simulink model "DR18E_Testpult"  (R2017a)
settings: Solver=ode1  StartTime=0.0  StopTime=Inf  FixedStep=0.001  RelTol=1e-3
PostLoadFcn:
  | , if any(exist('dsrtsu_mdlpostloadfcn', 'file') == [2, 3, 6]), try dsrtsu_mdlpostloadfcn('Execute', bdroot); catch fprintf('Error in PostLoadFcn (dsrtsu_mdlpostloadfcn) for model "%s":\n %s\n', bdroot, lasterr); end, end,
model workspace: external: MAT-File C:\Users\DeltaRacing\Documents\dSPACE\MABX_DR18E\Model\DR18E_MABX_Parameter.mat (data not in the file)
values from neighbouring files (symbols this model uses):
  am = 1/Ts    (= 1)    [DR18E_MABX_Parameter.m]
  bm = K/Ts    (= 0.05)    [DR18E_MABX_Parameter.m]
  cf = 41350    [DR18E_MABX_Parameter.m]
  cr = 41350    [DR18E_MABX_Parameter.m]
  Derating_HV_Battery_Kapa = 1    [DR18E_MABX_Parameter.m]
  Derating_Start_km = 16    [DR18E_MABX_Parameter.m]
  Drive_Mode = 0    [DR18E_MABX_Parameter.m]
  g = 1    [DR18E_MABX_Parameter.m]
  Gas_Modus = 2    [DR18E_MABX_Parameter.m]
  HV_Power_max = 80    [DR18E_MABX_Parameter.m]
  i_Getriebe = 3.3    [DR18E_MABX_Parameter.m]
  i_Lenkgetriebe = 4.32    [DR18E_MABX_Parameter.m]
  K_SET = 1    [DR18E_MABX_Parameter.m]
  Kapazitaet_HV_Battery_kWh = 6.6    [DR18E_MABX_Parameter.m]
  KW_T_Soll = 37    [DR18E_MABX_Parameter.m]
  lf = 1.2    [DR18E_MABX_Parameter.m]
  lr = 1.15    [DR18E_MABX_Parameter.m]
  m = mdriver + mvehicle    (= 310)    [DR18E_MABX_Parameter.m]
  M_max = 150    [DR18E_MABX_Parameter.m]
  Power_Limit_onoff = 0    [DR18E_MABX_Parameter.m]
  Reifenradius = 0.2351    [DR18E_MABX_Parameter.m]
  Strecke_Endu_km = 22    [DR18E_MABX_Parameter.m]
  TC_Decr_Gas = 0.00005    (= 5e-05)    [DR18E_MABX_Parameter.m]
  TC_Derivative = 0.4    [DR18E_MABX_Parameter.m]
  TC_Incr_Gas = 0.005    [DR18E_MABX_Parameter.m]
  TC_On = 0    [DR18E_MABX_Parameter.m]
  TC_Relay_Off = 0.065    [DR18E_MABX_Parameter.m]
  TC_Relay_On = 0.07    [DR18E_MABX_Parameter.m]
  TV_Mode = 2    [DR18E_MABX_Parameter.m]
  TV_On = 0    [DR18E_MABX_Parameter.m]
  TV_Override = 1    [DR18E_MABX_Parameter.m]
  y = 0.8    [DR18E_MABX_Parameter.m]
undefined symbols (not defined in the file or in its folder): D, DiscIntNeverNeededParam, I, K_OL, P
libraries: simulink x288, rtican x100, rtiusbflightreclib x40, rti1401lib_dio_type3 x10, simulink_extras x10, rti1401lib_adc_type4 x8, rti1401lib_II_base x7
(part 27 of 27)

== system DR18E_Testpult/Eingabe Fahrzeug/BMS/Voltage Stack 1-2/Voltage Stack 2/RX Timeout Detection2/Subsystem ==
  TXStatus : Inport
  Timeout : Inport  Port=2
  Constant : Constant
  Constant1 : Constant  Value=0
  Constant2 : Constant
  Constant3 : Constant  Value=0
  Delay : Delay  DelayLength=1  InitialCondition=0
  Relational Operator : RelationalOperator  Operator=>  OutDataTypeStr=boolean  RndMeth=Nearest
  Sum : Sum  Inputs=|++
  Switch : Switch  Criteria=u2 > Threshold
  Switch1 : Switch  Criteria=u2 > Threshold
  Rampe : Outport
  RX Timeout Error : Outport  Port=2
  wires:
  TXStatus/1 -> Switch/2
  Delay/1 -> Sum/2
  Constant/1 -> Sum/1
  Sum/1 -> Switch/3
  Switch/1 -> Delay/1, Relational Operator/1, Rampe/1
  Constant1/1 -> Switch/1
  Constant2/1 -> Switch1/1
  Constant3/1 -> Switch1/3
  Switch1/1 -> RX Timeout Error/1
  Relational Operator/1 -> Switch1/2
  Timeout/1 -> Relational Operator/2

== system DR18E_Testpult/Eingabe Fahrzeug/BMS/Voltage Stack 3-4/Voltage Stack 3/RX Timeout Detection/Subsystem ==
  TXStatus : Inport
  Timeout : Inport  Port=2
  Constant : Constant
  Constant1 : Constant  Value=0
  Constant2 : Constant
  Constant3 : Constant  Value=0
  Delay : Delay  DelayLength=1  InitialCondition=0
  Relational Operator : RelationalOperator  Operator=>  OutDataTypeStr=boolean  RndMeth=Nearest
  Sum : Sum  Inputs=|++
  Switch : Switch  Criteria=u2 > Threshold
  Switch1 : Switch  Criteria=u2 > Threshold
  Rampe : Outport
  RX Timeout Error : Outport  Port=2
  wires:
  TXStatus/1 -> Switch/2
  Delay/1 -> Sum/2
  Constant/1 -> Sum/1
  Sum/1 -> Switch/3
  Switch/1 -> Delay/1, Relational Operator/1, Rampe/1
  Constant1/1 -> Switch/1
  Constant2/1 -> Switch1/1
  Constant3/1 -> Switch1/3
  Switch1/1 -> RX Timeout Error/1
  Relational Operator/1 -> Switch1/2
  Timeout/1 -> Relational Operator/2

== system DR18E_Testpult/Eingabe Fahrzeug/BMS/Voltage Stack 3-4/Voltage Stack 3/RX Timeout Detection1/Subsystem ==
  TXStatus : Inport
  Timeout : Inport  Port=2
  Constant : Constant
  Constant1 : Constant  Value=0
  Constant2 : Constant
  Constant3 : Constant  Value=0
  Delay : Delay  DelayLength=1  InitialCondition=0
  Relational Operator : RelationalOperator  Operator=>  OutDataTypeStr=boolean  RndMeth=Nearest
  Sum : Sum  Inputs=|++
  Switch : Switch  Criteria=u2 > Threshold
  Switch1 : Switch  Criteria=u2 > Threshold
  Rampe : Outport
  RX Timeout Error : Outport  Port=2
  wires:
  TXStatus/1 -> Switch/2
  Delay/1 -> Sum/2
  Constant/1 -> Sum/1
  Sum/1 -> Switch/3
  Switch/1 -> Delay/1, Relational Operator/1, Rampe/1
  Constant1/1 -> Switch/1
  Constant2/1 -> Switch1/1
  Constant3/1 -> Switch1/3
  Switch1/1 -> RX Timeout Error/1
  Relational Operator/1 -> Switch1/2
  Timeout/1 -> Relational Operator/2

== system DR18E_Testpult/Eingabe Fahrzeug/BMS/Voltage Stack 3-4/Voltage Stack 3/RX Timeout Detection2/Subsystem ==
  TXStatus : Inport
  Timeout : Inport  Port=2
  Constant : Constant
  Constant1 : Constant  Value=0
  Constant2 : Constant
  Constant3 : Constant  Value=0
  Delay : Delay  DelayLength=1  InitialCondition=0
  Relational Operator : RelationalOperator  Operator=>  OutDataTypeStr=boolean  RndMeth=Nearest
  Sum : Sum  Inputs=|++
  Switch : Switch  Criteria=u2 > Threshold
  Switch1 : Switch  Criteria=u2 > Threshold
  Rampe : Outport
  RX Timeout Error : Outport  Port=2
  wires:
  TXStatus/1 -> Switch/2
  Delay/1 -> Sum/2
  Constant/1 -> Sum/1
  Sum/1 -> Switch/3
  Switch/1 -> Delay/1, Relational Operator/1, Rampe/1
  Constant1/1 -> Switch/1
  Constant2/1 -> Switch1/1
  Constant3/1 -> Switch1/3
  Switch1/1 -> RX Timeout Error/1
  Relational Operator/1 -> Switch1/2
  Timeout/1 -> Relational Operator/2

== system DR18E_Testpult/Eingabe Fahrzeug/BMS/Voltage Stack 3-4/Voltage Stack 4/RX Timeout Detection/Subsystem ==
  TXStatus : Inport
  Timeout : Inport  Port=2
  Constant : Constant
  Constant1 : Constant  Value=0
  Constant2 : Constant
  Constant3 : Constant  Value=0
  Delay : Delay  DelayLength=1  InitialCondition=0
  Relational Operator : RelationalOperator  Operator=>  OutDataTypeStr=boolean  RndMeth=Nearest
  Sum : Sum  Inputs=|++
  Switch : Switch  Criteria=u2 > Threshold
  Switch1 : Switch  Criteria=u2 > Threshold
  Rampe : Outport
  RX Timeout Error : Outport  Port=2
  wires:
  TXStatus/1 -> Switch/2
  Delay/1 -> Sum/2
  Constant/1 -> Sum/1
  Sum/1 -> Switch/3
  Switch/1 -> Delay/1, Relational Operator/1, Rampe/1
  Constant1/1 -> Switch/1
  Constant2/1 -> Switch1/1
  Constant3/1 -> Switch1/3
  Switch1/1 -> RX Timeout Error/1
  Relational Operator/1 -> Switch1/2
  Timeout/1 -> Relational Operator/2

== system DR18E_Testpult/Eingabe Fahrzeug/BMS/Voltage Stack 3-4/Voltage Stack 4/RX Timeout Detection1/Subsystem ==
  TXStatus : Inport
  Timeout : Inport  Port=2
  Constant : Constant
  Constant1 : Constant  Value=0
  Constant2 : Constant
  Constant3 : Constant  Value=0
  Delay : Delay  DelayLength=1  InitialCondition=0
  Relational Operator : RelationalOperator  Operator=>  OutDataTypeStr=boolean  RndMeth=Nearest
  Sum : Sum  Inputs=|++
  Switch : Switch  Criteria=u2 > Threshold
  Switch1 : Switch  Criteria=u2 > Threshold
  Rampe : Outport
  RX Timeout Error : Outport  Port=2
  wires:
  TXStatus/1 -> Switch/2
  Delay/1 -> Sum/2
  Constant/1 -> Sum/1
  Sum/1 -> Switch/3
  Switch/1 -> Delay/1, Relational Operator/1, Rampe/1
  Constant1/1 -> Switch/1
  Constant2/1 -> Switch1/1
  Constant3/1 -> Switch1/3
  Switch1/1 -> RX Timeout Error/1
  Relational Operator/1 -> Switch1/2
  Timeout/1 -> Relational Operator/2

== system DR18E_Testpult/Eingabe Fahrzeug/BMS/Voltage Stack 3-4/Voltage Stack 4/RX Timeout Detection2/Subsystem ==
  TXStatus : Inport
  Timeout : Inport  Port=2
  Constant : Constant
  Constant1 : Constant  Value=0
  Constant2 : Constant
  Constant3 : Constant  Value=0
  Delay : Delay  DelayLength=1  InitialCondition=0
  Relational Operator : RelationalOperator  Operator=>  OutDataTypeStr=boolean  RndMeth=Nearest
  Sum : Sum  Inputs=|++
  Switch : Switch  Criteria=u2 > Threshold
  Switch1 : Switch  Criteria=u2 > Threshold
  Rampe : Outport
  RX Timeout Error : Outport  Port=2
  wires:
  TXStatus/1 -> Switch/2
  Delay/1 -> Sum/2
  Constant/1 -> Sum/1
  Sum/1 -> Switch/3
  Switch/1 -> Delay/1, Relational Operator/1, Rampe/1
  Constant1/1 -> Switch/1
  Constant2/1 -> Switch1/1
  Constant3/1 -> Switch1/3
  Switch1/1 -> RX Timeout Error/1
  Relational Operator/1 -> Switch1/2
  Timeout/1 -> Relational Operator/2

== system DR18E_Testpult/Eingabe Fahrzeug/BMS/Voltage Stack 5-6/Voltage Stack 5/RX Timeout Detection/Subsystem ==
  TXStatus : Inport
  Timeout : Inport  Port=2
  Constant : Constant
  Constant1 : Constant  Value=0
  Constant2 : Constant
  Constant3 : Constant  Value=0
  Delay : Delay  DelayLength=1  InitialCondition=0
  Relational Operator : RelationalOperator  Operator=>  OutDataTypeStr=boolean  RndMeth=Nearest
  Sum : Sum  Inputs=|++
  Switch : Switch  Criteria=u2 > Threshold
  Switch1 : Switch  Criteria=u2 > Threshold
  Rampe : Outport
  RX Timeout Error : Outport  Port=2
  wires:
  TXStatus/1 -> Switch/2
  Delay/1 -> Sum/2
  Constant/1 -> Sum/1
  Sum/1 -> Switch/3
  Switch/1 -> Delay/1, Relational Operator/1, Rampe/1
  Constant1/1 -> Switch/1
  Constant2/1 -> Switch1/1
  Constant3/1 -> Switch1/3
  Switch1/1 -> RX Timeout Error/1
  Relational Operator/1 -> Switch1/2
  Timeout/1 -> Relational Operator/2

== system DR18E_Testpult/Eingabe Fahrzeug/BMS/Voltage Stack 5-6/Voltage Stack 5/RX Timeout Detection1/Subsystem ==
  TXStatus : Inport
  Timeout : Inport  Port=2
  Constant : Constant
  Constant1 : Constant  Value=0
  Constant2 : Constant
  Constant3 : Constant  Value=0
  Delay : Delay  DelayLength=1  InitialCondition=0
  Relational Operator : RelationalOperator  Operator=>  OutDataTypeStr=boolean  RndMeth=Nearest
  Sum : Sum  Inputs=|++
  Switch : Switch  Criteria=u2 > Threshold
  Switch1 : Switch  Criteria=u2 > Threshold
  Rampe : Outport
  RX Timeout Error : Outport  Port=2
  wires:
  TXStatus/1 -> Switch/2
  Delay/1 -> Sum/2
  Constant/1 -> Sum/1
  Sum/1 -> Switch/3
  Switch/1 -> Delay/1, Relational Operator/1, Rampe/1
  Constant1/1 -> Switch/1
  Constant2/1 -> Switch1/1
  Constant3/1 -> Switch1/3
  Switch1/1 -> RX Timeout Error/1
  Relational Operator/1 -> Switch1/2
  Timeout/1 -> Relational Operator/2

== system DR18E_Testpult/Eingabe Fahrzeug/BMS/Voltage Stack 5-6/Voltage Stack 5/RX Timeout Detection2/Subsystem ==
  TXStatus : Inport
  Timeout : Inport  Port=2
  Constant : Constant
  Constant1 : Constant  Value=0
  Constant2 : Constant
  Constant3 : Constant  Value=0
  Delay : Delay  DelayLength=1  InitialCondition=0
  Relational Operator : RelationalOperator  Operator=>  OutDataTypeStr=boolean  RndMeth=Nearest
  Sum : Sum  Inputs=|++
  Switch : Switch  Criteria=u2 > Threshold
  Switch1 : Switch  Criteria=u2 > Threshold
  Rampe : Outport
  RX Timeout Error : Outport  Port=2
  wires:
  TXStatus/1 -> Switch/2
  Delay/1 -> Sum/2
  Constant/1 -> Sum/1
  Sum/1 -> Switch/3
  Switch/1 -> Delay/1, Relational Operator/1, Rampe/1
  Constant1/1 -> Switch/1
  Constant2/1 -> Switch1/1
  Constant3/1 -> Switch1/3
  Switch1/1 -> RX Timeout Error/1
  Relational Operator/1 -> Switch1/2
  Timeout/1 -> Relational Operator/2

== system DR18E_Testpult/Eingabe Fahrzeug/BMS/Voltage Stack 5-6/Voltage Stack 6/RX Timeout Detection/Subsystem ==
  TXStatus : Inport
  Timeout : Inport  Port=2
  Constant : Constant
  Constant1 : Constant  Value=0
  Constant2 : Constant
  Constant3 : Constant  Value=0
  Delay : Delay  DelayLength=1  InitialCondition=0
  Relational Operator : RelationalOperator  Operator=>  OutDataTypeStr=boolean  RndMeth=Nearest
  Sum : Sum  Inputs=|++
  Switch : Switch  Criteria=u2 > Threshold
  Switch1 : Switch  Criteria=u2 > Threshold
  Rampe : Outport
  RX Timeout Error : Outport  Port=2
  wires:
  TXStatus/1 -> Switch/2
  Delay/1 -> Sum/2
  Constant/1 -> Sum/1
  Sum/1 -> Switch/3
  Switch/1 -> Delay/1, Relational Operator/1, Rampe/1
  Constant1/1 -> Switch/1
  Constant2/1 -> Switch1/1
  Constant3/1 -> Switch1/3
  Switch1/1 -> RX Timeout Error/1
  Relational Operator/1 -> Switch1/2
  Timeout/1 -> Relational Operator/2

== system DR18E_Testpult/Eingabe Fahrzeug/BMS/Voltage Stack 5-6/Voltage Stack 6/RX Timeout Detection1/Subsystem ==
  TXStatus : Inport
  Timeout : Inport  Port=2
  Constant : Constant
  Constant1 : Constant  Value=0
  Constant2 : Constant
  Constant3 : Constant  Value=0
  Delay : Delay  DelayLength=1  InitialCondition=0
  Relational Operator : RelationalOperator  Operator=>  OutDataTypeStr=boolean  RndMeth=Nearest
  Sum : Sum  Inputs=|++
  Switch : Switch  Criteria=u2 > Threshold
  Switch1 : Switch  Criteria=u2 > Threshold
  Rampe : Outport
  RX Timeout Error : Outport  Port=2
  wires:
  TXStatus/1 -> Switch/2
  Delay/1 -> Sum/2
  Constant/1 -> Sum/1
  Sum/1 -> Switch/3
  Switch/1 -> Delay/1, Relational Operator/1, Rampe/1
  Constant1/1 -> Switch/1
  Constant2/1 -> Switch1/1
  Constant3/1 -> Switch1/3
  Switch1/1 -> RX Timeout Error/1
  Relational Operator/1 -> Switch1/2
  Timeout/1 -> Relational Operator/2

== system DR18E_Testpult/Eingabe Fahrzeug/BMS/Voltage Stack 5-6/Voltage Stack 6/RX Timeout Detection2/Subsystem ==
  TXStatus : Inport
  Timeout : Inport  Port=2
  Constant : Constant
  Constant1 : Constant  Value=0
  Constant2 : Constant
  Constant3 : Constant  Value=0
  Delay : Delay  DelayLength=1  InitialCondition=0
  Relational Operator : RelationalOperator  Operator=>  OutDataTypeStr=boolean  RndMeth=Nearest
  Sum : Sum  Inputs=|++
  Switch : Switch  Criteria=u2 > Threshold
  Switch1 : Switch  Criteria=u2 > Threshold
  Rampe : Outport
  RX Timeout Error : Outport  Port=2
  wires:
  TXStatus/1 -> Switch/2
  Delay/1 -> Sum/2
  Constant/1 -> Sum/1
  Sum/1 -> Switch/3
  Switch/1 -> Delay/1, Relational Operator/1, Rampe/1
  Constant1/1 -> Switch/1
  Constant2/1 -> Switch1/1
  Constant3/1 -> Switch1/3
  Switch1/1 -> RX Timeout Error/1
  Relational Operator/1 -> Switch1/2
  Timeout/1 -> Relational Operator/2

== system DR18E_Testpult/Eingabe Fahrzeug/BMS/Voltage Stack 7-8/Voltage Stack 7/RX Timeout Detection/Subsystem ==
  TXStatus : Inport
  Timeout : Inport  Port=2
  Constant : Constant
  Constant1 : Constant  Value=0
  Constant2 : Constant
  Constant3 : Constant  Value=0
  Delay : Delay  DelayLength=1  InitialCondition=0
  Relational Operator : RelationalOperator  Operator=>  OutDataTypeStr=boolean  RndMeth=Nearest
  Sum : Sum  Inputs=|++
  Switch : Switch  Criteria=u2 > Threshold
  Switch1 : Switch  Criteria=u2 > Threshold
  Rampe : Outport
  RX Timeout Error : Outport  Port=2
  wires:
  TXStatus/1 -> Switch/2
  Delay/1 -> Sum/2
  Constant/1 -> Sum/1
  Sum/1 -> Switch/3
  Switch/1 -> Delay/1, Relational Operator/1, Rampe/1
  Constant1/1 -> Switch/1
  Constant2/1 -> Switch1/1
  Constant3/1 -> Switch1/3
  Switch1/1 -> RX Timeout Error/1
  Relational Operator/1 -> Switch1/2
  Timeout/1 -> Relational Operator/2

== system DR18E_Testpult/Eingabe Fahrzeug/BMS/Voltage Stack 7-8/Voltage Stack 7/RX Timeout Detection1/Subsystem ==
  TXStatus : Inport
  Timeout : Inport  Port=2
  Constant : Constant
  Constant1 : Constant  Value=0
  Constant2 : Constant
  Constant3 : Constant  Value=0
  Delay : Delay  DelayLength=1  InitialCondition=0
  Relational Operator : RelationalOperator  Operator=>  OutDataTypeStr=boolean  RndMeth=Nearest
  Sum : Sum  Inputs=|++
  Switch : Switch  Criteria=u2 > Threshold
  Switch1 : Switch  Criteria=u2 > Threshold
  Rampe : Outport
  RX Timeout Error : Outport  Port=2
  wires:
  TXStatus/1 -> Switch/2
  Delay/1 -> Sum/2
  Constant/1 -> Sum/1
  Sum/1 -> Switch/3
  Switch/1 -> Delay/1, Relational Operator/1, Rampe/1
  Constant1/1 -> Switch/1
  Constant2/1 -> Switch1/1
  Constant3/1 -> Switch1/3
  Switch1/1 -> RX Timeout Error/1
  Relational Operator/1 -> Switch1/2
  Timeout/1 -> Relational Operator/2

== system DR18E_Testpult/Eingabe Fahrzeug/BMS/Voltage Stack 7-8/Voltage Stack 7/RX Timeout Detection2/Subsystem ==
  TXStatus : Inport
  Timeout : Inport  Port=2
  Constant : Constant
  Constant1 : Constant  Value=0
  Constant2 : Constant
  Constant3 : Constant  Value=0
  Delay : Delay  DelayLength=1  InitialCondition=0
  Relational Operator : RelationalOperator  Operator=>  OutDataTypeStr=boolean  RndMeth=Nearest
  Sum : Sum  Inputs=|++
  Switch : Switch  Criteria=u2 > Threshold
  Switch1 : Switch  Criteria=u2 > Threshold
  Rampe : Outport
  RX Timeout Error : Outport  Port=2
  wires:
  TXStatus/1 -> Switch/2
  Delay/1 -> Sum/2
  Constant/1 -> Sum/1
  Sum/1 -> Switch/3
  Switch/1 -> Delay/1, Relational Operator/1, Rampe/1
  Constant1/1 -> Switch/1
  Constant2/1 -> Switch1/1
  Constant3/1 -> Switch1/3
  Switch1/1 -> RX Timeout Error/1
  Relational Operator/1 -> Switch1/2
  Timeout/1 -> Relational Operator/2

== system DR18E_Testpult/Eingabe Fahrzeug/BMS/Voltage Stack 7-8/Voltage Stack 8/RX Timeout Detection/Subsystem ==
  TXStatus : Inport
  Timeout : Inport  Port=2
  Constant : Constant
  Constant1 : Constant  Value=0
  Constant2 : Constant
  Constant3 : Constant  Value=0
  Delay : Delay  DelayLength=1  InitialCondition=0
  Relational Operator : RelationalOperator  Operator=>  OutDataTypeStr=boolean  RndMeth=Nearest
  Sum : Sum  Inputs=|++
  Switch : Switch  Criteria=u2 > Threshold
  Switch1 : Switch  Criteria=u2 > Threshold
  Rampe : Outport
  RX Timeout Error : Outport  Port=2
  wires:
  TXStatus/1 -> Switch/2
  Delay/1 -> Sum/2
  Constant/1 -> Sum/1
  Sum/1 -> Switch/3
  Switch/1 -> Delay/1, Relational Operator/1, Rampe/1
  Constant1/1 -> Switch/1
  Constant2/1 -> Switch1/1
  Constant3/1 -> Switch1/3
  Switch1/1 -> RX Timeout Error/1
  Relational Operator/1 -> Switch1/2
  Timeout/1 -> Relational Operator/2

== system DR18E_Testpult/Eingabe Fahrzeug/BMS/Voltage Stack 7-8/Voltage Stack 8/RX Timeout Detection1/Subsystem ==
  TXStatus : Inport
  Timeout : Inport  Port=2
  Constant : Constant
  Constant1 : Constant  Value=0
  Constant2 : Constant
  Constant3 : Constant  Value=0
  Delay : Delay  DelayLength=1  InitialCondition=0
  Relational Operator : RelationalOperator  Operator=>  OutDataTypeStr=boolean  RndMeth=Nearest
  Sum : Sum  Inputs=|++
  Switch : Switch  Criteria=u2 > Threshold
  Switch1 : Switch  Criteria=u2 > Threshold
  Rampe : Outport
  RX Timeout Error : Outport  Port=2
  wires:
  TXStatus/1 -> Switch/2
  Delay/1 -> Sum/2
  Constant/1 -> Sum/1
  Sum/1 -> Switch/3
  Switch/1 -> Delay/1, Relational Operator/1, Rampe/1
  Constant1/1 -> Switch/1
  Constant2/1 -> Switch1/1
  Constant3/1 -> Switch1/3
  Switch1/1 -> RX Timeout Error/1
  Relational Operator/1 -> Switch1/2
  Timeout/1 -> Relational Operator/2

== system DR18E_Testpult/Eingabe Fahrzeug/BMS/Voltage Stack 7-8/Voltage Stack 8/RX Timeout Detection2/Subsystem ==
  TXStatus : Inport
  Timeout : Inport  Port=2
  Constant : Constant
  Constant1 : Constant  Value=0
  Constant2 : Constant
  Constant3 : Constant  Value=0
  Delay : Delay  DelayLength=1  InitialCondition=0
  Relational Operator : RelationalOperator  Operator=>  OutDataTypeStr=boolean  RndMeth=Nearest
  Sum : Sum  Inputs=|++
  Switch : Switch  Criteria=u2 > Threshold
  Switch1 : Switch  Criteria=u2 > Threshold
  Rampe : Outport
  RX Timeout Error : Outport  Port=2
  wires:
  TXStatus/1 -> Switch/2
  Delay/1 -> Sum/2
  Constant/1 -> Sum/1
  Sum/1 -> Switch/3
  Switch/1 -> Delay/1, Relational Operator/1, Rampe/1
  Constant1/1 -> Switch/1
  Constant2/1 -> Switch1/1
  Constant3/1 -> Switch1/3
  Switch1/1 -> RX Timeout Error/1
  Relational Operator/1 -> Switch1/2
  Timeout/1 -> Relational Operator/2

== system DR18E_Testpult/Eingabe Fahrzeug/Inverter Feedback Messages/Istwerte Umrichter 1 empfangen /Drehzahl/PT1 Discrete2/Subsystem ==
  T : Inport
  Constant : Constant
  Constant2 : Constant
  Divide : Product  Inputs=*/
  Divide1 : Product  Inputs=*/
  Sum : Sum  Inputs=|++
  Weighted Sample Time : SampleTimeMath  TsampMathOp=Ts Only
  T* : Outport
  wires:
  Divide1/1 -> Sum/1
  Constant2/1 -> Sum/2
  T/1 -> Divide1/1
  Sum/1 -> Divide/2
  Constant/1 -> Divide/1
  Weighted Sample Time/1 -> Divide1/2
  Divide/1 -> T*/1

== system DR18E_Testpult/Eingabe Fahrzeug/Inverter Feedback Messages/Istwerte Umrichter 2 empfangen/Drehzahl/PT1 Discrete2/Subsystem ==
  T : Inport
  Constant : Constant
  Constant2 : Constant
  Divide : Product  Inputs=*/
  Divide1 : Product  Inputs=*/
  Sum : Sum  Inputs=|++
  Weighted Sample Time : SampleTimeMath  TsampMathOp=Ts Only
  T* : Outport
  wires:
  Divide1/1 -> Sum/1
  Constant2/1 -> Sum/2
  T/1 -> Divide1/1
  Sum/1 -> Divide/2
  Constant/1 -> Divide/1
  Weighted Sample Time/1 -> Divide1/2
  Divide/1 -> T*/1

== system DR18E_Testpult/Eingabe Fahrzeug/MicroAutoBox/AI/Umrechnung Widerstand - Temperatur NTC/PT1 Discrete1/Subsystem ==
  T : Inport
  Constant : Constant
  Constant2 : Constant
  Divide : Product  Inputs=*/
  Divide1 : Product  Inputs=*/
  Sum : Sum  Inputs=|++
  Weighted Sample Time : SampleTimeMath  TsampMathOp=Ts Only
  T* : Outport
  wires:
  Divide1/1 -> Sum/1
  Constant2/1 -> Sum/2
  T/1 -> Divide1/1
  Sum/1 -> Divide/2
  Constant/1 -> Divide/1
  Weighted Sample Time/1 -> Divide1/2
  Divide/1 -> T*/1

== system DR18E_Testpult/Eingabe Fahrzeug/MicroAutoBox/AI/Umrechnung Widerstand - Temperatur NTC1/PT1 Discrete1/Subsystem ==
  T : Inport
  Constant : Constant
  Constant2 : Constant
  Divide : Product  Inputs=*/
  Divide1 : Product  Inputs=*/
  Sum : Sum  Inputs=|++
  Weighted Sample Time : SampleTimeMath  TsampMathOp=Ts Only
  T* : Outport
  wires:
  Divide1/1 -> Sum/1
  Constant2/1 -> Sum/2
  T/1 -> Divide1/1
  Sum/1 -> Divide/2
  Constant/1 -> Divide/1
  Weighted Sample Time/1 -> Divide1/2
  Divide/1 -> T*/1

== stateflow chart DR18E_Testpult/Verarbeitung/Vehicle State Machine/Fahrzeugsteuerung ==
  settings: updateMethod=DISCRETE  sampleTime=1e-3
  state Init
    en: O_Sicherheitskreis_Enable = 0;
    settings: description=|
        | Umrichter Initialisierung
        | 
        | Parametrierung der beiden Umrichter, damit Ist-Werte zyklisch gesendet werden.
    state UmrichterInit
      en: O_Inverter_TX_Mode = 1; //TX Modus: Initialisierung
      state initEntry
        en: O_State = 10;
      state U_init
        en: O_State = 11;
        en: O_U1Init_Reg = I_vecU1config_TXRegister[i];
        en: O_U1Init_Zeit = I_vecU1config_TXZeiten[i];
        en: O_U2Init_Reg = I_vecU2config_TXRegister[i];
        en: O_U2Init_Zeit = I_vecU2config_TXZeiten[i] ;
      note: For-Schleife
          | über alle
          | 8 Configs
      state wait
        en: O_State = 12;
      state CANTimeoutInit
        /*en: O_U1_RegID = 208; //0xD0
        en: O_U2_RegID = 208; //0xD0
        en: O_U1_Value32 = 1000; //Timeout in ms
        en: O_U2_Value32 = 1000; //Timeout in ms*/
        en: O_Inverter_TX_Mode = 2;
        //Universal TX Mode
        ex: O_U1_RegID = 0;
        ex: O_U1_RegID = 0;
      (default) -> initEntry
      initEntry -> (junction 759) : after(5,sec)
      (junction 759) -> (junction 211) : {i = 0;}
      (junction 211) -> U_init [order 1] : [i < 8]
      (junction 222) -> (junction 211) : {i++;}
      (junction 211) -> CANTimeoutInit [order 2]
      U_init -> wait : after(0.01,sec)
      wait -> (junction 222) : after(0.1,sec)
    state Boards_Init
      en: en: O_Inverter_TX_Mode = 2;
      //Universal TX Mode
      en: Board_Init_ok = 1;
      en: O_InvertersTXActive = 1;
      en: O_State = 16;
      en: O_coolingEnable = 0;
    state Check_Safety
      state Error_In_Flash
        en: O_AMSIMDFlash = 1;
        en: en: O_State = 18.1;
      state Safety_Error2
        en: O_ErrorNr = 6;
        en: O_State = 17.7;
        exit: e_Error;
      state Error_In_Flash_Reset
        en: O_AMSIMDFlash = 0;
        en: O_State = 18.2;
      state Safety_Error3
        en: O_ErrorNr = 7;
        en: O_State = 17.8;
        exit: e_Error;
      note: ERROR
      state Safety_Error
        en: O_ErrorNr = 2;
        en: O_State = 17.1;
        exit: e_Error;
      state Safety_Error1
        en: O_ErrorNr = 1;
        en: O_State = 17.2;
        exit: e_Error;
      state Safety_Error4
        en: O_ErrorNr = 3;
        en: O_State = 17.3;
        exit: e_Error;
      state Safety_Error5
        en: O_ErrorNr = 4;
        en: O_State = 17.4;
        exit: e_Error;
      state Safety_Error6
        en: O_ErrorNr = 5;
        en: O_State = 17.5;
        exit: e_Error;
      state Safety_Error7
        en: O_ErrorNr = 8;
        en: O_State = 17.6;
        exit: e_Error;
      state Safety_Error_Reset
        en: O_ErrorNr = 0;
        en: O_AMSIMDFlash = 0;
        en: O_State = 19;
        exit: e_Error;
      (junction 673) -> (junction 671) : after(0.2,sec)
      (default) -> (junction 671)
      Init.Check_Safety.Safety_Error2 -> Init.Check_Safety.Error_In_Flash
      (junction 671) -> Init.Check_Safety.Safety_Error2 [order 2] : [A_AMS]
      (junction 671) -> (junction 672) [order 1] : [!A_AMS]
      (junction 672) -> Init.Check_Safety.Safety_Error3 [order 1] : [A_IMD]
      Init.Check_Safety.Safety_Error3 -> Init.Check_Safety.Error_In_Flash
      (junction 672) -> (junction 674) [order 2] : [!A_IMD]
      Init.Check_Safety.Error_In_Flash_Reset -> (junction 673)
      Init.Check_Safety.Safety_Error -> (junction 673)
      Init.Check_Safety.Safety_Error4 -> (junction 673)
      Init.Check_Safety.Safety_Error7 -> (junction 673)
      Init.Check_Safety.Safety_Error6 -> (junction 673)
      Init.Check_Safety.Safety_Error5 -> (junction 673)
      Init.Check_Safety.Safety_Error1 -> (junction 673)
      Init.Check_Safety.Error_In_Flash -> Init.Check_Safety.Error_In_Flash_Reset : [I_AMS_IMD_Reset]
      (junction 674) -> Init.Check_Safety.Safety_Error [order 2] : [A_BRAKE_OVERTRAVEL]
      (junction 674) -> (junction 675) [order 1] : [!A_BRAKE_OVERTRAVEL]
      (junction 675) -> Init.Check_Safety.Safety_Error1 [order 1] : [A_BPD]
      (junction 675) -> (junction 676) [order 2] : [!A_BPD]
      (junction 676) -> Init.Check_Safety.Safety_Error4 [order 1] : [A_NOT_COCKPIT]
      (junction 676) -> (junction 677) [order 2] : [!A_NOT_COCKPIT]
      (junction 677) -> Init.Check_Safety.Safety_Error5 [order 1] : [A_NOT_LINKS]
      (junction 677) -> (junction 678) [order 2] : [!A_NOT_LINKS]
      (junction 678) -> Init.Check_Safety.Safety_Error6 [order 1] : [A_NOT_RECHTS]
      (junction 678) -> (junction 679) [order 2] : [!A_NOT_RECHTS]
      (junction 679) -> Init.Check_Safety.Safety_Error7 [order 1] : [A_HVD]
      (junction 679) -> Init.Check_Safety.Safety_Error_Reset [order 2] : [!A_HVD]
    state Blink_Start_Button
      en: O_State = 20;
      en: Init_complete = 1;
    CANTimeoutInit -> Boards_Init : after(0.1,sec)
        | /*Umrichter Init Complete*/
    (default) -> UmrichterInit
    Boards_Init -> Check_Safety
    Init.Check_Safety.Safety_Error_Reset -> Blink_Start_Button
  note: Systeminitialisierung
  state Idle
    en: O_Sicherheitskreis_Enable = 0;
    en: O_State = 21;
    en: O_fBlink_Start = 2;
    settings: description=|
        | Idle-Modus
        | 
        | GLVS ist aktiv
        | TS ist inaktiv
        | 
        | Grundzustand der Fahrzeugsteuerung. Alle Antriebssysteme sind dekativiert, AIRs sind geöffnet.
        | Verlassen des Zustands durch Drücken der Start-Taste bei gleichzeitigem Betätigen des Bremspedals.
        | 
        | In diesen Zustand wird aus allen Zuständen zurückgekehrt, sobald der Sicherheitskreis anspricht.
  state TS_init
    settings: description=|
        | TS-Init Modus
        | 
        | Initialisierung des Tractive Systems.
        | Das heißt:
        | -Precharge
        | -Prüfen ob AIRs geschlossen sind und Ziel-Ladespannung des Zwischenkreises erreicht ist
        | 
        | Zustand wird verlassen, wenn Precharge abgeschlossen, AIRs geschlossen und Ziel-Spannung erreicht ist
    note: Sicherheitskreis geschlossen
        | und Entladerelais geöffnet
    state Precharge
      du: O_fBlink_Start = 0;
      state Precharge_Prepare
        en: O_Precharge_Enable = 1;
        en: O_State = 22;
      state Precharge_Start
        en: O_Sicherheitskreis_Enable = 1;
        en: O_State = 23;
        //du: e_clearPowervoltage;
      note: Precharge startet!
      state AIR_Error4
        en: O_ErrorNr = 36;
        en: O_State = 24.1;
        exit: e_Error;
      state AIR_Error
        en: O_ErrorNr = 31;
        en: O_State = 24.2;
        exit: e_Error;
      state AIR_Error1
        en: O_ErrorNr = 32;
        en: O_State = 24.3;
        exit: e_Error;
      state Precharge_TimeError
        en: O_ErrorNr = 33;
        en: O_State = 25;
        exit: e_Error;
      state Precharge_Done
        en: O_Precharge_Enable = 0;
        en: O_ErrorNr = 0;
        en: O_State = 26;
        exit: e_Error;
      state AIR_Disable
        en: O_Sicherheitskreis_Enable = 0;
        en: O_Precharge_Enable = 0;
        en: O_State = 24.4;
      state AIR_Error2
        en: O_ErrorNr = 34;
        en: O_State = 27.1;
        exit: e_Error;
      state AIR_Error3
        en: O_ErrorNr = 35;
        en: O_State = 27.2;
        exit: e_Error;
      state AIR_Error5
        en: O_ErrorNr = 37;
        en: O_State = 27.3;
        exit: e_Error;
      note: Precharge erledigt, nun
          | Prechargerelais öffnen.
          | Pluspol  AIRs schließen
          | automatisch durch Verriegelung
          | gegen Precharge Relais
      (default) -> Precharge_Prepare
      Precharge_Prepare -> Precharge_Start : after(0.1,sec)
      Precharge_Start -> (junction 291) [order 2] : [false]
          | //after(0.5,sec)
      Precharge_Start -> (junction 290) [order 1] : //[AIR_L & AIR_Rminus]
      (junction 291) -> AIR_Error4 [order 3] : //beide Relais schalten nicht
          | [!AIR_L]
      (junction 291) -> AIR_Error [order 1] : [!AIR_L]
      (junction 291) -> AIR_Error1 [order 2] : [AIR_L]
      (junction 290) -> Precharge_Done [order 2] : //EV4.12.1
          | [I_U_Zwischenkreis >= (0.90*I_U_Batt)]
      (junction 290) -> Precharge_TimeError [order 1] : //Zu lange PrechargeZeit
          | after(15,sec)
      AIR_Error1 -> (junction 299)
      AIR_Error4 -> (junction 299)
      AIR_Error -> (junction 299)
      Precharge_TimeError -> (junction 299)
      Precharge_Done -> (junction 386) [order 1] : [false]
          | //after(0.5,sec)
      (junction 299) -> AIR_Disable
      AIR_Error5 -> (junction 299)
      AIR_Error3 -> (junction 299)
      AIR_Error2 -> (junction 299)
      (junction 386) -> AIR_Error2 [order 1] : [AIR_R]
      (junction 386) -> AIR_Error5 [order 3] : //beide AIRs schließen nicht
          | [!AIR_R]
      (junction 386) -> AIR_Error3 [order 2] : [!AIR_R]
    note: TODO:
        | Error Handling
    state ClearPowervoltageError
      /*en: O_U1_RegID = 143; //0x8F
      en: O_U2_RegID = 143; //0x8F
      en: O_U1_Value32 = 0;
      en: O_U2_Value32 = 0;
      en: O_Inverter_TX_Mode = 2; //Universal TX Mode
      ex: O_U1_RegID = 0;
      ex: O_U1_RegID = 0;*/
    (default) -> Precharge
    Precharge_Done -> ClearPowervoltageError [order 2] : //Precharge OK
        | [AIR_R]
  state Check_Safety1
    en: O_Sicherheitskreis_Enable = 0;
    en: O_Precharge_Enable = 0
    en: O_fBlink_Start = 0;
    state Error_In_Flash
      en: O_AMSIMDFlash = 1;
      en: en: O_State = 48.1;
    state Safety_Error2
      en: O_ErrorNr = 6;
      en: O_State = 47.7;
      exit: e_Error;
    state Error_In_Flash_Reset
      en: O_AMSIMDFlash = 0;
      en: O_State = 48.2;
    state Safety_Error3
      en: O_ErrorNr = 7;
      en: O_State = 47.8;
      exit: e_Error;
    state Safety_Error
      en: O_ErrorNr = 2;
      en: O_State = 47.1;
      exit: e_Error;
    state Safety_Error1
      en: O_ErrorNr = 1;
      en: O_State = 47.2;
      exit: e_Error;
    state Safety_Error4
      en: O_ErrorNr = 3;
      en: O_State = 47.3;
      exit: e_Error;
    state Safety_Error5
      en: O_ErrorNr = 4;
      en: O_State = 47.4;
      exit: e_Error;
    state Safety_Error6
      en: O_ErrorNr = 5;
      en: O_State = 47.5;
      exit: e_Error;
    state Safety_Error7
      en: O_ErrorNr = 8;
      en: O_State = 47.6;
      exit: e_Error;
    state Safety_Error_Reset
      en: O_ErrorNr = 0;
      en: O_State = 49;
      exit: e_Error;
    note: Sicherheitskreis ok
    (default) -> (junction 617)
    Check_Safety1.Safety_Error2 -> Check_Safety1.Error_In_Flash
    (junction 617) -> Check_Safety1.Safety_Error2 [order 2] : [A_AMS]
    (junction 617) -> (junction 618) [order 1] : [!A_AMS]
    (junction 618) -> Check_Safety1.Safety_Error3 [order 1] : [A_IMD]
    Check_Safety1.Safety_Error3 -> Check_Safety1.Error_In_Flash
    (junction 618) -> (junction 619) [order 2] : [!A_IMD]
    Check_Safety1.Error_In_Flash_Reset -> (junction 625)
    Check_Safety1.Error_In_Flash -> Check_Safety1.Error_In_Flash_Reset : //[I_AMS_IMD_Reset]
    (junction 619) -> Check_Safety1.Safety_Error [order 2] : [A_BRAKE_OVERTRAVEL]
    Check_Safety1.Safety_Error -> (junction 625)
    (junction 619) -> (junction 620) [order 1] : [!A_BRAKE_OVERTRAVEL]
    (junction 620) -> Check_Safety1.Safety_Error1 [order 1] : [A_BPD]
    Check_Safety1.Safety_Error1 -> (junction 625)
    (junction 620) -> (junction 621) [order 2] : [!A_BPD]
    (junction 621) -> Check_Safety1.Safety_Error4 [order 1] : [A_NOT_COCKPIT]
    (junction 621) -> (junction 622) [order 2] : [!A_NOT_COCKPIT]
    Check_Safety1.Safety_Error4 -> (junction 625)
    (junction 622) -> Check_Safety1.Safety_Error5 [order 1] : [A_NOT_LINKS]
    Check_Safety1.Safety_Error5 -> (junction 625)
    (junction 622) -> (junction 623) [order 2] : [!A_NOT_LINKS]
    (junction 623) -> Check_Safety1.Safety_Error6 [order 1] : [A_NOT_RECHTS]
    (junction 623) -> (junction 624) [order 2] : [!A_NOT_RECHTS]
    Check_Safety1.Safety_Error6 -> (junction 625)
    (junction 624) -> Check_Safety1.Safety_Error7 [order 1] : [A_HVD]
    Check_Safety1.Safety_Error7 -> (junction 625)
    (junction 624) -> Check_Safety1.Safety_Error_Reset [order 2] : [!A_HVD]
    Check_Safety1.Safety_Error_Reset -> (junction 625)
  note: Was hat
      | Sicherheitskreis
      | ausgelöst?
  state TS_ready
    en: O_fBlink_Start = 10;
    en: O_State = 40;
    en: O_SoundEnable = 1;
    ex: O_Inverter_TX_Mode = 3; //TX Mode: Torque
    settings: description=|
        | TS ready Modus
        | 
        | Tractive System ist fertig initialisiert und wartet auf Freischaltung durch den Fahrer per Start-Button.
  state Sound
    en: O_fBlink_Start = 0;
    en: O_State = 41;
    en: O_SpeakerEnable = 1;
    exit: O_SpeakerEnable= 0;
    exit: O_coolingEnable= 1;
    settings: description=|
        | Sound-Modus
        | 
        | Tractive Sound ausgeben
    note: Zum abspielen muss ein Impuls
        | am jeweiligen Kanal erzeugt werden
    state PlaySound_Pulse
      en: O_SoundPlayChannel = 1;
    state PlaySound_Pulse1
      en: O_SoundPlayChannel = 0;
    (default) -> PlaySound_Pulse
    PlaySound_Pulse -> PlaySound_Pulse1 : after(0.5,sec)
  state TS_active
    en: O_fBlink_Start = 0;
    en: O_State = 50;
    //en: O_Inverter_TX_Mode = 3; //TX Mode: Torque
    en: O_InverterFRE = 1; //Inverter Freigabe
    settings: description=|
        | TS_active Modus
        | 
        | Das Antriebssystem befindet sich im betriebsbereiten Zustand.
        | 
        | Zustand wird verlassen, sobald ein Fehler auftritt (immer in Shutdown-Modus zum sicheren Herunterfahren)
    state AccelerationMode
    state BasicMode
      //Torque Vectoring nicht aktiv
      du: O_enableTorqueVectoring = 0;
      //Schlupfregelung nicht aktiv
      du: O_enableTractionControl = 0;
      //Gaspedalstellung = Drehmomentsollwert, rechts und links gleich
      //Pmax per Fernzugriff begrenzbar
      du: O_enableRemotePmax = 1;
    state SkidpadMode
    state EnduranceMode
    AccelerationMode -> EnduranceMode [order 2] : [I_Drive_Mode == 3]
    AccelerationMode -> SkidpadMode [order 1] : [I_Drive_Mode == 2]
    EnduranceMode -> AccelerationMode [order 3] : [I_Drive_Mode == 1]
    SkidpadMode -> AccelerationMode [order 2] : [I_Drive_Mode == 1]
    BasicMode -> AccelerationMode [order 2] : [I_Drive_Mode == 1]
    AccelerationMode -> BasicMode [order 3] : [I_Drive_Mode == 0]
    (default) -> BasicMode : //Default: Basic
    BasicMode -> EnduranceMode [order 3] : [I_Drive_Mode == 3]
    SkidpadMode -> BasicMode [order 1] : [I_Drive_Mode == 0]
    EnduranceMode -> BasicMode [order 2] : [I_Drive_Mode == 0]
    BasicMode -> SkidpadMode [order 1] : [I_Drive_Mode == 2]
    SkidpadMode -> EnduranceMode [order 3] : [I_Drive_Mode == 3]
    EnduranceMode -> SkidpadMode [order 1] : [I_Drive_Mode == 2]
  state SafetyShutdown
    settings: description=|
        | Shutdown-Modus
        | 
        | Sicheres herunterfahren des Antriebssystems innerhalb von 250ms
    state TorqueToZero
      en: O_State = 70.1;
      en: O_U1_RegID = 144; //0x90
      en: O_U2_RegID = 144; //0x90
      en: O_U1_Value32 = 0;
      en: O_U2_Value32 = 0;
      en: O_Inverter_TX_Mode = 2;
      //Universal TX Mode
      ex: O_U1_RegID = 0;
      ex: O_U1_RegID = 0;
    state LockInverters
      en: O_State = 70.2;
      en: O_InverterFRE = 0;
    state OpenShutdown
      en: O_State = 70.3;
      en: O_Sicherheitskreis_Enable = 0;
    (default) -> SafetyShutdown.TorqueToZero
    SafetyShutdown.TorqueToZero -> SafetyShutdown.LockInverters : after(0.05,sec)
    SafetyShutdown.LockInverters -> SafetyShutdown.OpenShutdown : after(0.05,sec)
  note: Systemleistung
      | sicher reduzieren
  state NormalShutdown
    settings: description=|
        | Shutdown-Modus
        | 
        | Sicheres herunterfahren des Antriebssystems innerhalb von 250ms
    state TorqueToZero
      en: O_State = 70.1;
      en: O_U1_RegID = 144; //0x90
      en: O_U2_RegID = 144; //0x90
      en: O_U1_Value32 = 0;
      en: O_U2_Value32 = 0;
      en: O_Inverter_TX_Mode = 2;
      //Universal TX Mode
      ex: O_U1_RegID = 0;
      ex: O_U1_RegID = 0;
    state LockInverters
      en: O_State = 70.2;
      en: O_InverterFRE = 0;
    state OpenShutdown
      en: O_State = 70.3;
      en: O_Sicherheitskreis_Enable = 0;
    state Shutdown_Message
      en: O_ErrorNr = 81;
      en: O_State = 70.4;
      exit: e_Error;
    (default) -> NormalShutdown.TorqueToZero
    NormalShutdown.TorqueToZero -> NormalShutdown.LockInverters : after(0.05,sec)
    NormalShutdown.LockInverters -> NormalShutdown.OpenShutdown : after(0.05,sec)
    NormalShutdown.OpenShutdown -> Shutdown_Message
  PlaySound_Pulse1 -> TS_active : after(1,sec)
  Shutdown_Message -> Idle
  Blink_Start_Button -> Idle : [Init_complete]
  (junction 625) -> Idle : //Fehlerquelle gefunden und gemeldet
  (default) -> Init
  SafetyShutdown.OpenShutdown -> (junction 11)
  Idle -> TS_init : [I_StartButton & !I_Sicherheitskreis &  I_Bremse_bin]
  ClearPowervoltageError -> TS_ready : after(0.1,sec)
  AIR_Disable -> (junction 11) : //Precharge Error
      | after(0.1,sec)
  TS_init -> (junction 11) : [I_Sicherheitskreis]
  (junction 11) -> Check_Safety1
  TS_ready -> (junction 11) [order 1] : [I_Sicherheitskreis | !AIR_L  | !AIR_R]
  TS_ready -> Sound [order 2] : [I_StartButton & I_Bremse_bin]
  TS_active -> TS_ready [order 1] : [false]
      | /*Platzhalter
      | für Rückkehr in
      | leistungslosen Zustand*/
  Sound -> SafetyShutdown : [I_Sicherheitskreis]
  TS_active -> SafetyShutdown [order 3] : [I_Sicherheitskreis | !AIR_L | !AIR_R]
  TS_active -> NormalShutdown [order 2] : [I_StartButton]
  data: i local int8 =1; Board_Init_ok local boolean; I_StartButton input; Shutdown_complete local boolean =0; Init_complete local boolean; O_TS_sound output int16; I_Sicherheitskreis input; AIR_L input; AIR_R input; O_U1_RegID output; O_U2_RegID output; O_U2_Value32 output; O_U1_Value32 output; I_vecU1config_TXRegister input size=8; I_vecU1config_TXZeiten input size=8; I_vecU2config_TXRegister input size=8; I_vecU2config_TXZeiten input size=8; I_Dischg_Feedback input; A_BPD input; A_BRAKE_OVERTRAVEL input; A_NOT_COCKPIT input; A_NOT_LINKS input; A_NOT_RECHTS input; A_AMS input; A_IMD input; A_HVD input; O_Sicherheitskreis_Enable output boolean size=1; I_U_Zwischenkreis input double; I_U_Batt input double; O_Precharge_Enable output boolean; O_ErrorNr output size=1 =0; I_AMS_IMD_Reset input; O_fBlink_Start output double; O_State output double =0; O_enableTorqueVectoring output uint8 =0; O_enableTractionControl output uint8 =0; O_enableRemotePmax local uint8 =1; O_InverterFRE output double =0; O_TorqueEnable output double =0; O_InvertersTXActive output double =0; O_AMSIMDFlash output uint8 =0; O_U1Init_Reg output double; O_U1Init_Zeit output double; O_U2Init_Reg output double; O_U2Init_Zeit output double; O_Inverter_TX_Mode output uint16; O_SoundEnable output uint8; O_SoundPlayChannel output double; O_SpeakerEnable output double; O_coolingEnable output double =1; I_Drive_Mode input double; I_Bremse_bin input
  events: e_U1_TX output FUNCTION_CALL_EVENT; e_Error output EITHER_EDGE_EVENT; e_ACTIVE output EITHER_EDGE_EVENT; e_clearPowervoltage output EITHER_EDGE_EVENT

== stateflow chart DR18E_Testpult/Ausgabe/Inverter TX/TX Mode Management ==
  state Init
    en: O_Init = 1;
    ex: O_Init = 0;
  state Off
  state Universal
    en: O_Universal = 1;
    ex: O_Universal = 0;
  state Torque
    en: O_Torque = 1;
    ex: O_Torque = 0;
  Init -> Universal [order 2] : [TX_Mode == 2]
  Init -> Torque [order 1] : [TX_Mode == 3]
  Universal -> Init [order 3] : [TX_Mode == 1]
  Torque -> Init [order 3] : [TX_Mode == 1]
  Off -> Init [order 3] : [TX_Mode == 1]
  Init -> Off [order 3] : [TX_Mode == 0]
  (default) -> Off
  Off -> Universal [order 2] : [TX_Mode == 2]
  Off -> Torque [order 1] : [TX_Mode == 3]
  Universal -> Off [order 1] : [TX_Mode == 0]
  Torque -> Off [order 1] : [TX_Mode == 0]
  Torque -> Universal [order 2] : [TX_Mode == 2]
  Universal -> Torque [order 2] : [TX_Mode == 3]
  data: TX_Mode input uint16; O_Universal output boolean =0; O_Init output boolean =0; O_Torque output boolean =0
